simulink model "hysteresis1"  (R2023b)
settings: Solver=FixedStepAuto  StartTime=0.0  StopTime=86400  FixedStep=1  RelTol=1  AbsTol=1
undefined symbols (not defined in the file): IAU, WMM2020
libraries: aerolibtransform2 x3, vrlib x2, shared6dof x1, aerolibgravity2 x1
settings Model: SimulationMode=accelerator  Creator=mikey  LastModifiedBy=mikey
settings SolverCC: AutoScaleAbsTol=off
settings DebuggingCC: SignalInfNanChecking=warning

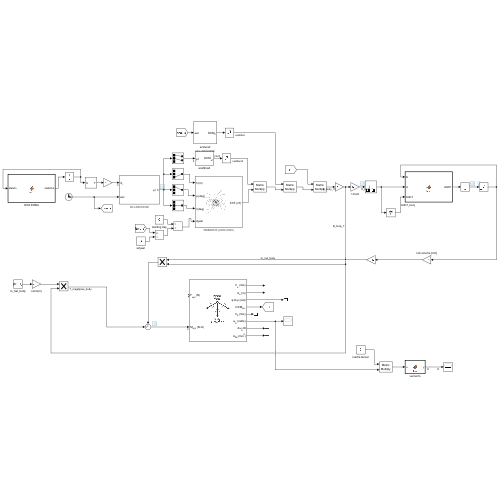
[thumbnail: Simulink's stored preview of the top-level diagram]
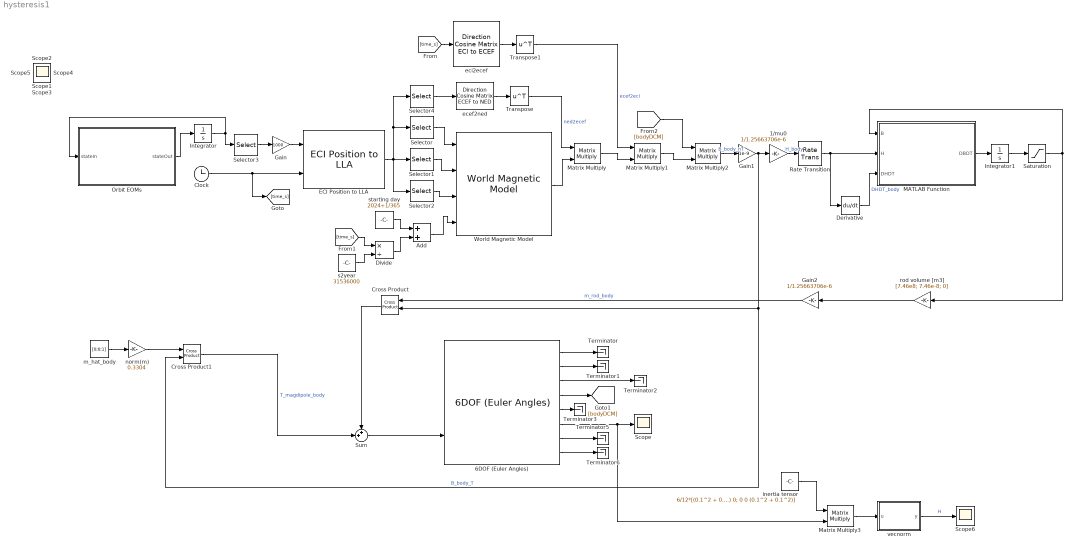
== system hysteresis1 ==
  1/mu0 : Gain  Gain=1/1.25663706e-6
  6DOF (Euler Angles) : shared6dof/6DOF (Euler Angles)  units=Metric (MKS)  mtype=Fixed  rep=Quaternion  xme_0=[0 0 0]  Vm_0=[0 0 0]  eul_0=[0 0 0]  pm_0=[deg2rad(2) deg2rad(2) deg2rad(2)]  mass_0=6  mass_e=0.5  mass_f=2.0  inertia=6/12*[(0.1^2 + 0.3^2) 0 0; 0 (0.1^2 + 0.3^2) 0; 0 0 (0.1^2 + 0.1^2)]  inertia_e=eye(3)  inertia_f=2*eye(3)  k_quat=1.0  vre_flag=on  abi_flag=off  aMode=0  xme_statename=''  Vm_statename=''  eul_statename=''  quat_statename=''  pm_statename=''  mass_statename=''
  Add : Sum
  Clock : Clock
  Cross Product : vrlib/Utilities/Cross Product
  Cross Product1 : vrlib/Utilities/Cross Product
  Derivative : Derivative
  Divide : Product  Inputs=*/
  ECI Position to LLA : aerolibtransform2/ECI Position to LLA  red=IAU-2000/2006  year=2024  month=January  day=1  hour=0  min=0  sec=0  deltaT=Sec  errorflag=Error  extraparamflag=off  eunits=Metric (MKS)  earthmodel=WGS84  flat=1/298.257223563  eqradius=6378137
      settings: AttributesFormatString=%<red>
  Gain : Gain  Gain=1000
  Gain1 : Gain  Gain=1e-9
  Gain2 : Gain  Gain=1/1.25663706e-6
  Integrator : Integrator  InitialCondition=[6778;0;0;0;sqrt(398600/6778);0]
  Integrator1 : Integrator
  MATLAB Function : MATLAB Function  TreatAsAtomicUnit=on
  Matrix Multiply{,1..3} (4 alike) : Product  Multiplication=Matrix(*)
  Orbit EOMs : MATLAB Function  TreatAsAtomicUnit=on
  Rate Transition : RateTransition  OutPortSampleTimeOpt=Inherit
  Saturation : Saturate  UpperLimit=0.73  LowerLimit=-0.73
  Scope{,1..6} (7 alike) : Scope
  Selector : Selector  InputPortWidth=3  IndexOptions=Index vector (dialog)  Indices=3  OutputSizes=1
  Selector1 : Selector  InputPortWidth=3  IndexOptions=Index vector (dialog)  Indices=1  OutputSizes=1
  Selector2 : Selector  InputPortWidth=3  IndexOptions=Index vector (dialog)  Indices=2  OutputSizes=1
  Selector3 : Selector  InputPortWidth=6  IndexOptions=Index vector (dialog)  Indices=[1 2 3]  OutputSizes=1
  Selector4 : Selector  InputPortWidth=3  IndexOptions=Index vector (dialog)  Indices=[1 2]  OutputSizes=1
  Sum : Sum  Inputs=++|
  Terminator{,1..3,5..6} (6 alike) : Terminator
  Transpose : Math  Operator=transpose
  Transpose1 : Math  Operator=transpose
  World Magnetic Model : aerolibgravity2/World Magnetic Model  model=WMM2020 (2020-2025)  customFile='WMM2020.COF'  units=Metric (MKS)  time_in=on  month=January  day=1  year=2025  action=Error  h_out=off  dec_out=off  inc_out=off  ti_out=off
  ecef2ned : aerolibtransform2/Direction Cosine Matrix ECEF to NED
  eci2ecef : aerolibtransform2/Direction Cosine Matrix ECI to ECEF  red=IAU-2000/2006  year=2013  month=January  day=1  hour=0  min=0  sec=0  deltaT=Sec  errorflag=Error  extraparamflag=off
      settings: AttributesFormatString=%<red>
  inertia tensor : Constant  Value=6/12*[(0.1^2 + 0.3^2) 0 0; 0 (0.1^2 + 0.3^2) 0; 0 0 (0.1^2 + 0.1^2)]
  m_hat_body : Constant  Value=[0;0;1]
  norm(m) : Gain  Gain=0.3304
  rod volume [m3] : Gain  Gain=[7.46e8; 7.46e-8; 0]  ParamDataTypeStr=Inherit: Same as input
  s2year : Constant  Value=31536000
  starting day : Constant  Value=2024+1/365
  vecnorm : MATLAB Function  TreatAsAtomicUnit=on
  wires:
  Integrator/1 -> Selector3/1, Orbit EOMs/1(stateIn)
  Orbit EOMs/1(stateOut) -> Integrator/1
  ECI Position to LLA/1 -> Selector4/1, Selector/1, Selector2/1, Selector1/1
  Selector3/1 -> Gain/1
  Clock/1 -> ECI Position to LLA/2, [time_s]
  Selector1/1 -> World Magnetic Model/2
  Selector2/1 -> World Magnetic Model/3
  Selector/1 -> World Magnetic Model/1
  Gain/1 -> ECI Position to LLA/1
  ecef2ned/1 -> Transpose/1
  Selector4/1 -> ecef2ned/1
  Transpose/1 -> Matrix Multiply/1  "ned2ecef"
  World Magnetic Model/1 -> Matrix Multiply/2
  [time_s] -> eci2ecef/1
  eci2ecef/1 -> Transpose1/1
  Matrix Multiply/1 -> Matrix Multiply1/2
  Transpose1/1 -> Matrix Multiply1/1  "ecef2eci"
  [time_s] -> Divide/1
  s2year/1 -> Divide/2
  Divide/1 -> Add/2
  starting day/1 -> Add/1
  Add/1 -> World Magnetic Model/4
  m_hat_body/1 -> norm(m)/1
  6DOF (Euler Angles)/4 -> [bodyDCM]
  [bodyDCM] -> Matrix Multiply2/1
  Matrix Multiply1/1 -> Matrix Multiply2/2
  Matrix Multiply2/1 -> Gain1/1  "B_body_nT"
  norm(m)/1 -> Cross Product1/1
  Cross Product1/1 -> Sum/2  "T_magdipole_body"
  6DOF (Euler Angles)/1 -> Terminator/1
  6DOF (Euler Angles)/2 -> Terminator1/1
  6DOF (Euler Angles)/3 -> Terminator2/1
  6DOF (Euler Angles)/5 -> Terminator3/1
  6DOF (Euler Angles)/6 -> Matrix Multiply3/2, Scope/1
  6DOF (Euler Angles)/7 -> Terminator5/1
  6DOF (Euler Angles)/8 -> Terminator6/1
  MATLAB Function/1(DBDT) -> Integrator1/1
  Integrator1/1 -> Saturation/1
  Derivative/1 -> MATLAB Function/3(DHDT)  "DHDT_body"
  Gain2/1 -> Cross Product/1  "m_rod_body"
  rod volume [m3]/1 -> Gain2/1
  Gain1/1 -> 1/mu0/1, Cross Product/2, Cross Product1/2  "B_body_T"
  Saturation/1 -> rod volume [m3]/1, MATLAB Function/1(B)
  1/mu0/1 -> Rate Transition/1  "H_body"
  Rate Transition/1 -> Derivative/1, MATLAB Function/2(H)
  Sum/1 -> 6DOF (Euler Angles)/2
  Cross Product/1 -> Sum/1
  inertia tensor/1 -> Matrix Multiply3/1
  vecnorm/1(y) -> Scope6/1  "H"
  Matrix Multiply3/1 -> vecnorm/1(u)

== matlab function hysteresis1/MATLAB Function ==
  data: B input; DBDT output; H input; DHDT input
function DBDT = fcn(B, H, DHDT)
%#codegen
mu0 = 4*pi*1e-7; 
Bsx = 0.73;  % saturation flux density Tesla
Brx = 0.35;  % remanence, Tesla
Hcx = 1.59;  % coercive force A/m

k = 0.6;
p = 4.75;
q0 = 0.0885;

HL = tan(pi.*B./2./Bsx)./k - Hcx;

BP = 2 .* k .* Bsx/pi .* cos(pi*B/2/Bsx)*2;

F = (H-HL)/2/Hcx;

for i =1:3
    if(DHDT(i)<0)
        F(i) = 1-F(i);
    end
end


Q = q0 + (1-q0).*F.*p;

DBDT = Q.*BP.*DHDT;

== matlab function hysteresis1/Orbit EOMs ==
  data: stateOut output; stateIn input
function stateOut  = fcn(stateIn)

muEarth = 398600;

x = stateIn(1);
y = stateIn(2);
z = stateIn(3);

dx = stateIn(4);
dy = stateIn(5);
dz = stateIn(6);

r = norm([x y z]);

ddx = -muEarth*x/r^3;
ddy = -muEarth*y/r^3;
ddz = -muEarth*z/r^3;

stateOut = [dx; dy; dz; ddx; ddy; ddz];

== matlab function hysteresis1/vecnorm ==
  data: u input; y output
function y = fcn(u)

y = vecnorm(u;
